simulink model "SolarMicroinverterModelAnalogControl_230V"  (Simulink 8.4)
settings: Solver=ode5  StartTime=0.0  StopTime=0.042  FixedStep=1e-7  RelTol=1e-3
libraries: simulink x2
settings Model: Creator=I14724  LastModifiedBy=ilyas  ParamWorkspaceSource=ReferencedWorkspace  TunableVars=Ts  TunableVarsStorageClass=Auto
settings OptimizationCC: InitFltsAndDblsToZero=on

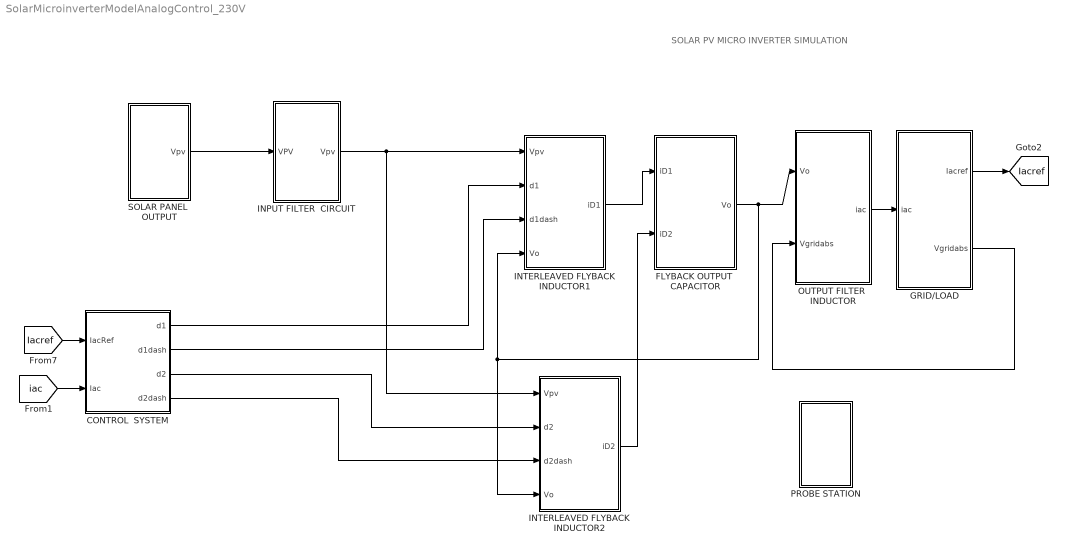
== system SolarMicroinverterModelAnalogControl_230V ==
  note: SOLAR PV MICRO INVERTER SIMULATION
  " CONTROL  SYSTEM" : Subsystem
  FLYBACK OUTPUT  CAPACITOR : Subsystem
  GRID/LOAD : Subsystem
  INPUT FILTER  CIRCUIT : Subsystem
  INTERLEAVED FLYBACK INDUCTOR1 : Subsystem
  INTERLEAVED FLYBACK INDUCTOR2 : Subsystem
  OUTPUT FILTER  INDUCTOR : Subsystem
  PROBE STATION : Subsystem
  SOLAR PANEL  OUTPUT : Subsystem
  tag scope: Iacref=global
  wires:
  INTERLEAVED FLYBACK INDUCTOR1/1(iD1) -> FLYBACK OUTPUT  CAPACITOR/1(iD1)
  FLYBACK OUTPUT  CAPACITOR/1(Vo) -> OUTPUT FILTER  INDUCTOR/1(Vo), INTERLEAVED FLYBACK INDUCTOR2/4(Vo), INTERLEAVED FLYBACK INDUCTOR1/4(Vo)
  OUTPUT FILTER  INDUCTOR/1(iac) -> GRID/LOAD/1(iac)
  GRID/LOAD/2(Vgridabs) -> OUTPUT FILTER  INDUCTOR/2(Vgridabs)
  GRID/LOAD/1(Iacref) -> [Iacref]
  SOLAR PANEL  OUTPUT/1(Vpv) -> INPUT FILTER  CIRCUIT/1(VPV)
  [Iacref] -> " CONTROL  SYSTEM"/1(IacRef)
  [iac] -> " CONTROL  SYSTEM"/2(Iac)
  " CONTROL  SYSTEM"/1(d1) -> INTERLEAVED FLYBACK INDUCTOR1/2(d1)
  " CONTROL  SYSTEM"/2(d1dash) -> INTERLEAVED FLYBACK INDUCTOR1/3(d1dash)
  INPUT FILTER  CIRCUIT/1(Vpv) -> INTERLEAVED FLYBACK INDUCTOR2/1(Vpv), INTERLEAVED FLYBACK INDUCTOR1/1(Vpv)
  " CONTROL  SYSTEM"/3(d2) -> INTERLEAVED FLYBACK INDUCTOR2/2(d2)
  " CONTROL  SYSTEM"/4(d2dash) -> INTERLEAVED FLYBACK INDUCTOR2/3(d2dash)
  INTERLEAVED FLYBACK INDUCTOR2/1(iD2) -> FLYBACK OUTPUT  CAPACITOR/2(iD2)

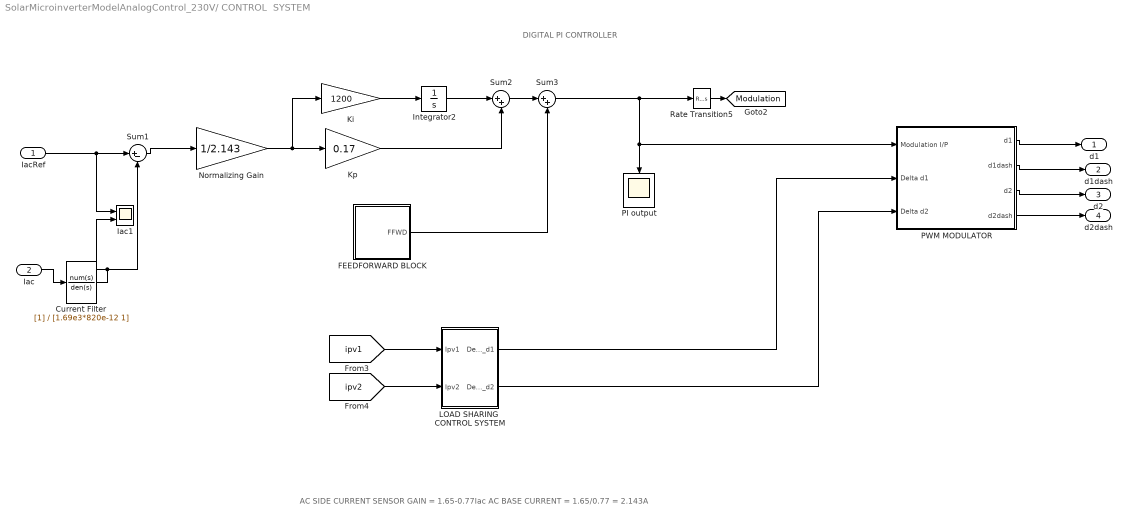
== system SolarMicroinverterModelAnalogControl_230V/ CONTROL  SYSTEM ==
  note: DIGITAL PI CONTROLLER
  note: AC SIDE CURRENT SENSOR GAIN = 1.65-0.77Iac
      | AC BASE CURRENT = 1.65/0.77 = 2.143A
  IacRef : Inport
  Iac : Inport  Port=2
  Current Filter : TransferFcn  Denominator=[1.69e3*820e-12 1]
  FEEDFORWARD BLOCK : Subsystem
  Iac1 : Scope  NumInputPorts=2
      settings: YMin=-5.5~-5.5  YMax=5.5~5.5  SaveName=ScopeData24
  Integrator2 : Integrator
  Ki : Gain  Gain=1200
  Kp : Gain  Gain=0.17
  LOAD SHARING  CONTROL SYSTEM : Subsystem
  Normalizing Gain : Gain  Gain=1/2.143
  PI output : Scope
      settings: TimeRange=0.01  YMin=0.15  YMax=0.5  SaveName=ScopeData15
  PWM MODULATOR : Subsystem
  Rate Transition5 : RateTransition  OutPortSampleTimeOpt=Inherit
  Sum1 : Sum  Inputs=|+-
  Sum2 : Sum  Inputs=|++
  Sum3 : Sum  Inputs=|++
  d1 : Outport
  d1dash : Outport  Port=2
  d2 : Outport  Port=3
  d2dash : Outport  Port=4
  tag scope: Modulation=global
  wires:
  IacRef/1 -> Sum1/1, Iac1/1
  PWM MODULATOR/1(d1) -> d1/1
  PWM MODULATOR/2(d1dash) -> d1dash/1
  Iac/1 -> Current Filter/1
  PWM MODULATOR/3(d2) -> d2/1
  PWM MODULATOR/4(d2dash) -> d2dash/1
  [ipv1] -> LOAD SHARING  CONTROL SYSTEM/1(Ipv1)
  [ipv2] -> LOAD SHARING  CONTROL SYSTEM/2(Ipv2)
  LOAD SHARING  CONTROL SYSTEM/1(Delta_d1) -> PWM MODULATOR/2(Delta d1)
  Rate Transition5/1 -> [Modulation]
  Sum1/1 -> Normalizing Gain/1
  Ki/1 -> Integrator2/1
  Normalizing Gain/1 -> Kp/1, Ki/1
  Sum2/1 -> Sum3/1
  Sum3/1 -> PI output/1, PWM MODULATOR/1(Modulation I/P), Rate Transition5/1
  Integrator2/1 -> Sum2/1
  Kp/1 -> Sum2/2
  FEEDFORWARD BLOCK/1(FFWD) -> Sum3/2
  LOAD SHARING  CONTROL SYSTEM/2(Delta_d2) -> PWM MODULATOR/3(Delta d2)
  Current Filter/1 -> Iac1/2, Sum1/2

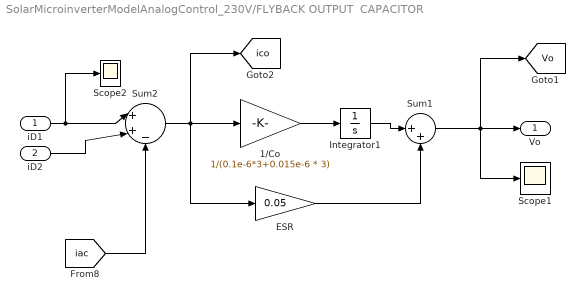
== system SolarMicroinverterModelAnalogControl_230V/FLYBACK OUTPUT  CAPACITOR ==
  iD1 : Inport
  iD2 : Inport  Port=2
  1/Co : Gain  Gain=1/(0.1e-6*3+0.015e-6 * 3)
  ESR : Gain  Gain=0.05
  Integrator1 : Integrator
  Scope1 : Scope
      settings: YMin=-25  YMax=350
  Scope2 : Scope
      settings: YMin=0  YMax=8  SaveName=ScopeData2
  Sum1 : Sum  Inputs=|++
  Sum2 : Sum  Inputs=|++-
  Vo : Outport
  tag scope: Vo=global, ico=global
  wires:
  1/Co/1 -> Integrator1/1
  Sum2/1 -> [ico], 1/Co/1, ESR/1
  Integrator1/1 -> Sum1/1
  Sum1/1 -> Vo/1, [Vo], Scope1/1
  ESR/1 -> Sum1/2
  iD1/1 -> Sum2/1, Scope2/1
  iD2/1 -> Sum2/2
  [iac] -> Sum2/3

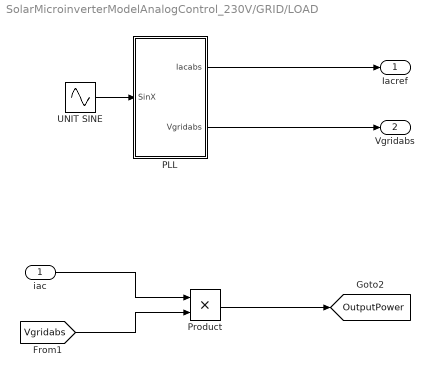
== system SolarMicroinverterModelAnalogControl_230V/GRID/LOAD ==
  iac : Inport
  PLL : Subsystem
  Product : Product  RndMeth=Zero
  UNIT SINE : Sin  Frequency=2*pi*60  SampleTime=0
  Iacref : Outport
  Vgridabs : Outport  Port=2
  tag scope: OutputPower=global
  wires:
  UNIT SINE/1 -> PLL/1(SinX)
  iac/1 -> Product/1
  Product/1 -> [OutputPower]
  [Vgridabs] -> Product/2
  PLL/1(Iacabs) -> Iacref/1
  PLL/2(Vgridabs) -> Vgridabs/1

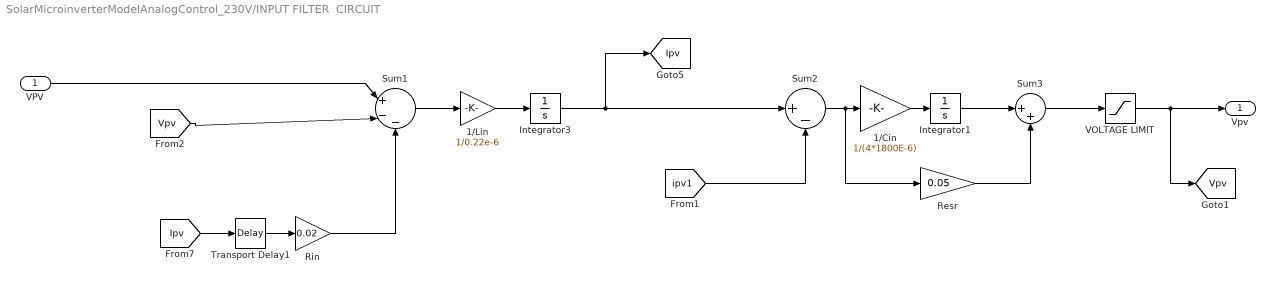
== system SolarMicroinverterModelAnalogControl_230V/INPUT FILTER  CIRCUIT ==
  VPV : Inport
  1/Cin : Gain  Gain=1/(4*1800E-6)
  1/Lin : Gain  Gain=1/0.22e-6
  Integrator1 : Integrator
  Integrator3 : Integrator
  Resr : Gain  Gain=0.05
  Rin : Gain  Gain=0.02
  Sum1 : Sum  Inputs=|+--
  Sum2 : Sum  Inputs=|+-
  Sum3 : Sum  Inputs=|++
  Transport Delay1 : TransportDelay  DelayTime=1e-7
  VOLTAGE LIMIT : Saturate  UpperLimit=100  LowerLimit=0
  Vpv : Outport
  tag scope: Ipv=global, Vpv=global
  wires:
  [ipv1] -> Sum2/2
  Integrator3/1 -> [Ipv], Sum2/1
  [Vpv] -> Sum1/2
  VPV/1 -> Sum1/1
  Rin/1 -> Sum1/3
  Transport Delay1/1 -> Rin/1
  [Ipv] -> Transport Delay1/1
  1/Lin/1 -> Integrator3/1
  Sum1/1 -> 1/Lin/1
  Sum2/1 -> 1/Cin/1, Resr/1
  1/Cin/1 -> Integrator1/1
  VOLTAGE LIMIT/1 -> Vpv/1, [Vpv]
  Integrator1/1 -> Sum3/1
  Sum3/1 -> VOLTAGE LIMIT/1
  Resr/1 -> Sum3/2

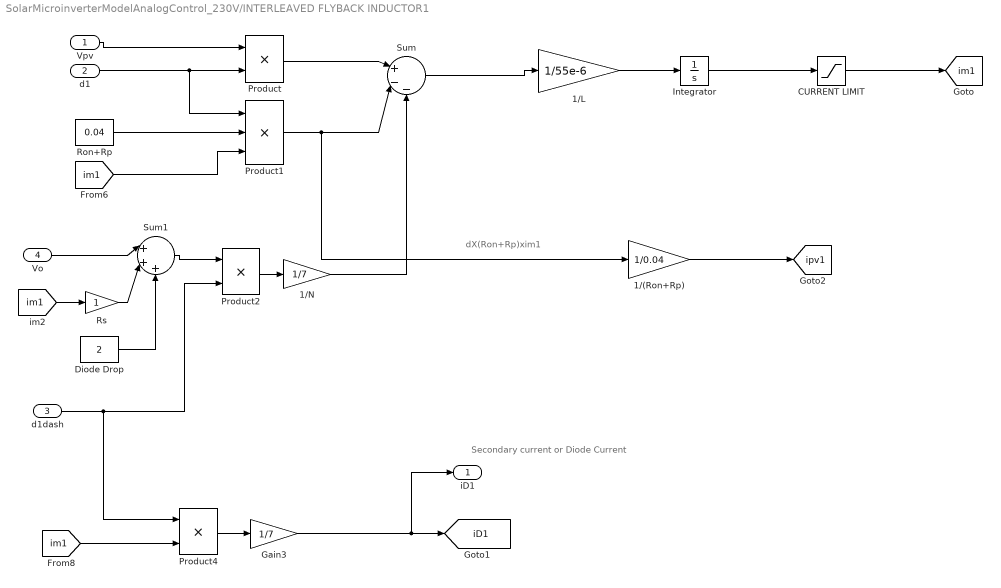
== system SolarMicroinverterModelAnalogControl_230V/INTERLEAVED FLYBACK INDUCTOR1 ==
  note: Secondary current or Diode Current
  note: dX(Ron+Rp)xim1
  Vpv : Inport
  d1 : Inport  Port=2
  d1dash : Inport  Port=3
  Vo : Inport  Port=4
  1/(Ron+Rp) : Gain  Gain=1/0.04
  1/L : Gain  Gain=1/55e-6
  1/N : Gain  Gain=1/7
  CURRENT LIMIT : Saturate  UpperLimit=200  LowerLimit=-1
  Diode Drop : Constant  Value=2
  Gain3 : Gain  Gain=1/7
  Integrator : Integrator
  Product : Product  RndMeth=Zero
  Product1 : Product  Inputs=3  RndMeth=Zero
  Product2 : Product  RndMeth=Zero
  Product4 : Product  RndMeth=Zero
  Ron+Rp : Constant  Value=0.04
  Rs : Gain
  Sum : Sum  Inputs=|+--
  Sum1 : Sum  Inputs=|+++
  iD1 : Outport
  tag scope: iD1=global, im1=global, ipv1=global
  wires:
  Integrator/1 -> CURRENT LIMIT/1
  1/N/1 -> Sum/3
  Product2/1 -> 1/N/1
  Sum1/1 -> Product2/1
  Product1/1 -> Sum/2, 1/(Ron+Rp)/1
  Product/1 -> Sum/1
  d1/1 -> Product/2, Product1/1
  Vpv/1 -> Product/1
  1/L/1 -> Integrator/1
  Sum/1 -> 1/L/1
  CURRENT LIMIT/1 -> [im1]
  [im1] -> Product4/2
  Gain3/1 -> [iD1], iD1/1
  Ron+Rp/1 -> Product1/2
  [im1] -> Product1/3
  Product4/1 -> Gain3/1
  Vo/1 -> Sum1/1
  d1dash/1 -> Product2/2, Product4/1
  1/(Ron+Rp)/1 -> [ipv1]
  [im1] -> Rs/1
  Diode Drop/1 -> Sum1/3
  Rs/1 -> Sum1/2

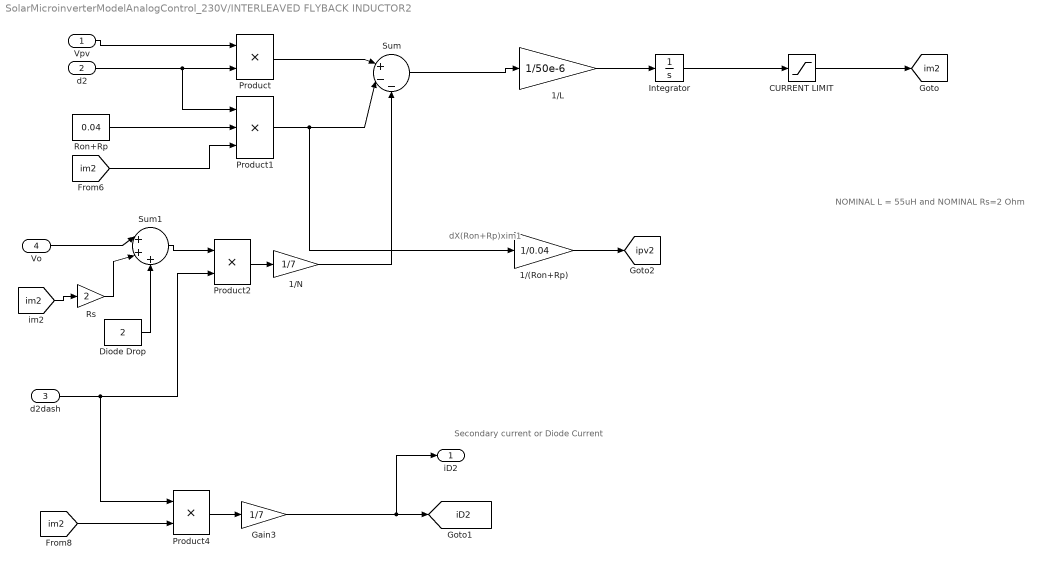
== system SolarMicroinverterModelAnalogControl_230V/INTERLEAVED FLYBACK INDUCTOR2 ==
  note: dX(Ron+Rp)xim1
  note: Secondary current or Diode Current
  note: NOMINAL L = 55uH and NOMINAL Rs=2 Ohm
  Vpv : Inport
  d2 : Inport  Port=2
  d2dash : Inport  Port=3
  Vo : Inport  Port=4
  1/(Ron+Rp) : Gain  Gain=1/0.04
  1/L : Gain  Gain=1/50e-6
  1/N : Gain  Gain=1/7
  CURRENT LIMIT : Saturate  UpperLimit=200  LowerLimit=-1
  Diode Drop : Constant  Value=2
  Gain3 : Gain  Gain=1/7
  Integrator : Integrator
  Product : Product  RndMeth=Zero
  Product1 : Product  Inputs=3  RndMeth=Zero
  Product2 : Product  RndMeth=Zero
  Product4 : Product  RndMeth=Zero
  Ron+Rp : Constant  Value=0.04
  Rs : Gain  Gain=2
  Sum : Sum  Inputs=|+--
  Sum1 : Sum  Inputs=|+++
  iD2 : Outport
  tag scope: iD2=global, im2=global, ipv2=global
  wires:
  1/(Ron+Rp)/1 -> [ipv2]
  d2dash/1 -> Product4/1, Product2/2
  Vo/1 -> Sum1/1
  Product4/1 -> Gain3/1
  [im2] -> Product1/3
  Ron+Rp/1 -> Product1/2
  Gain3/1 -> iD2/1, [iD2]
  [im2] -> Product4/2
  CURRENT LIMIT/1 -> [im2]
  Sum/1 -> 1/L/1
  1/L/1 -> Integrator/1
  Vpv/1 -> Product/1
  d2/1 -> Product1/1, Product/2
  Product/1 -> Sum/1
  Product1/1 -> 1/(Ron+Rp)/1, Sum/2
  [im2] -> Rs/1
  Sum1/1 -> Product2/1
  Product2/1 -> 1/N/1
  1/N/1 -> Sum/3
  Integrator/1 -> CURRENT LIMIT/1
  Rs/1 -> Sum1/2
  Diode Drop/1 -> Sum1/3

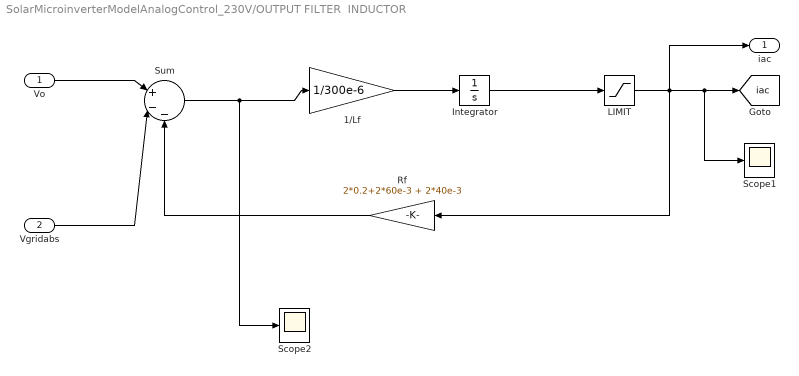
== system SolarMicroinverterModelAnalogControl_230V/OUTPUT FILTER  INDUCTOR ==
  Vo : Inport
  Vgridabs : Inport  Port=2
  " LIMIT" : Saturate  UpperLimit=10  LowerLimit=-0.4
  1/Lf : Gain  Gain=1/300e-6
  Integrator : Integrator
  Rf : Gain  Gain=2*0.2+2*60e-3 + 2*40e-3
  Scope1 : Scope
      settings: YMin=-0.2  YMax=1.2  SaveName=ScopeData8
  Scope2 : Scope
      settings: YMin=-3  YMax=3  SaveName=ScopeData13
  Sum : Sum  Inputs=|+--
  iac : Outport
  tag scope: iac=global
  wires:
  Vgridabs/1 -> Sum/2
  Integrator/1 -> " LIMIT"/1
  Vo/1 -> Sum/1
  1/Lf/1 -> Integrator/1
  Sum/1 -> 1/Lf/1, Scope2/1
  " LIMIT"/1 -> iac/1, Rf/1, [iac], Scope1/1
  Rf/1 -> Sum/3

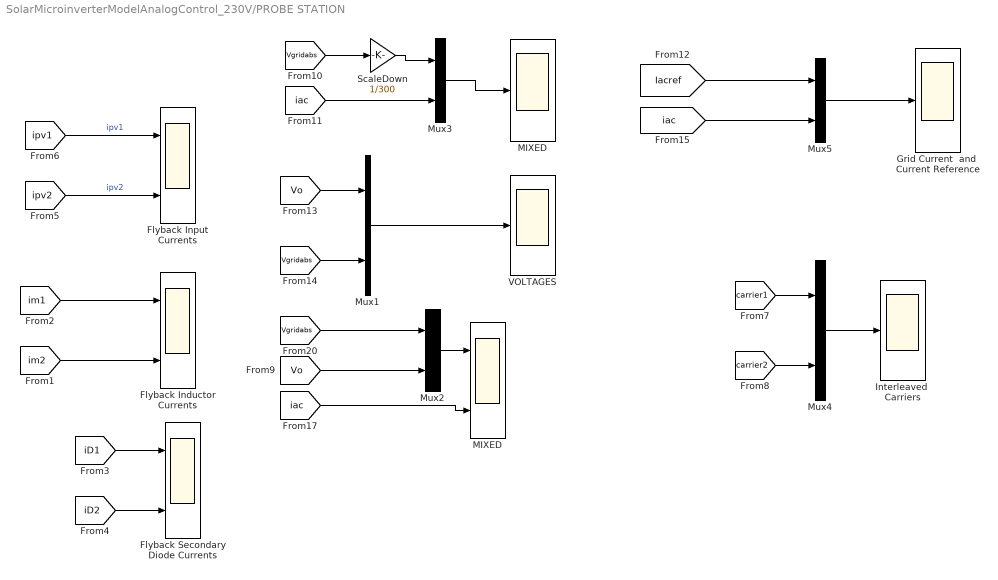
== system SolarMicroinverterModelAnalogControl_230V/PROBE STATION ==
  Flyback Inductor Currents : Scope  NumInputPorts=2
      settings: YMin=280~1.025  YMax=345~1.325
  Flyback Input Currents : Scope  NumInputPorts=2
      settings: YMin=280~1.025  YMax=345~1.325
  Flyback Secondary Diode Currents : Scope  NumInputPorts=2
      settings: YMin=280~1.025  YMax=345~1.325  SaveName=ScopeData2
  Grid Current  and  Current Reference : Scope
      settings: TimeRange=0.03  YMin=0.9  YMax=1.275  SaveName=ScopeData30
  Interleaved  Carriers : Scope
      settings: YMin=0  YMax=1  SaveName=ScopeData6
  MIXED : Scope
      settings: YMin=0.675  YMax=1.2  SaveName=ScopeData27
  "MIXED " : Scope  NumInputPorts=2
      settings: YMin=280~1.025  YMax=345~1.325  SaveName=ScopeData10
  Mux{1..5} (5 alike) : Mux  Inputs=2
  ScaleDown : Gain  Gain=1/300
  "VOLTAGES " : Scope
      settings: YMin=-1000  YMax=1500  SaveName=ScopeData9
  wires:
  [Vo] -> Mux1/1
  [Vgridabs] -> Mux1/2
  Mux1/1 -> "VOLTAGES "/1
  Mux2/1 -> "MIXED "/1
  [Vgridabs] -> Mux2/1
  [Vo] -> Mux2/2
  [iac] -> "MIXED "/2
  [carrier1] -> Mux4/1
  Mux4/1 -> Interleaved  Carriers/1
  [carrier2] -> Mux4/2
  Mux5/1 -> Grid Current  and  Current Reference/1
  [Iacref] -> Mux5/1
  [iac] -> Mux5/2
  [ipv1] -> Flyback Input Currents/1  "ipv1"
  [ipv2] -> Flyback Input Currents/2  "ipv2"
  [im1] -> Flyback Inductor Currents/1
  [im2] -> Flyback Inductor Currents/2
  [iD1] -> Flyback Secondary Diode Currents/1
  [iD2] -> Flyback Secondary Diode Currents/2
  Mux3/1 -> MIXED/1
  [Vgridabs] -> ScaleDown/1
  [iac] -> Mux3/2
  ScaleDown/1 -> Mux3/1

== system SolarMicroinverterModelAnalogControl_230V/SOLAR PANEL  OUTPUT ==
  Vmpp : Constant  Value=36
  Vpv : Outport
  tag scope: VPV=global
  wires:
  Vmpp/1 -> [VPV], Vpv/1

== system SolarMicroinverterModelAnalogControl_230V/ CONTROL  SYSTEM/FEEDFORWARD BLOCK ==
  Divide : Product  Inputs=*/
  Sum4 : Sum  Inputs=|++
  TURNS1 : Gain  Gain=7
  FFWD : Outport
  wires:
  [Vo] -> Sum4/1
  [Vpv] -> TURNS1/1
  [Vo] -> Divide/1
  Sum4/1 -> Divide/2
  TURNS1/1 -> Sum4/2
  Divide/1 -> FFWD/1

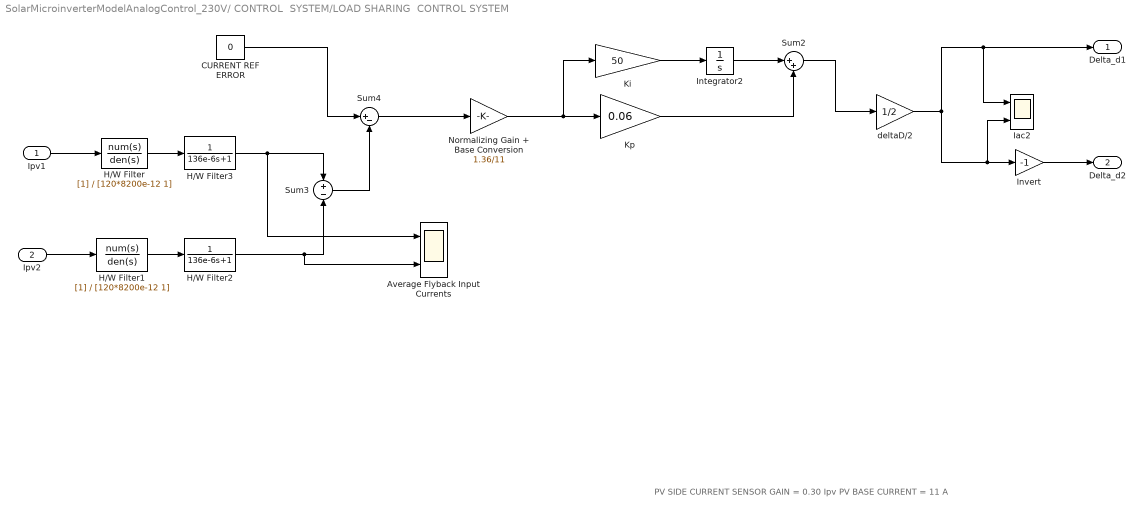
== system SolarMicroinverterModelAnalogControl_230V/ CONTROL  SYSTEM/LOAD SHARING  CONTROL SYSTEM ==
  note: PV SIDE CURRENT SENSOR GAIN = 0.30 Ipv
      | PV BASE CURRENT =  11 A
  Ipv1 : Inport
  Ipv2 : Inport  Port=2
  Average Flyback Input Currents : Scope  NumInputPorts=2
      settings: TimeRange=0.03  YMin=2.8~2.7  YMax=4.9~5  SaveName=ScopeData3
  CURRENT REF ERROR : Constant  Value=0
  H/W Filter : TransferFcn  Denominator=[120*8200e-12 1]
  H/W Filter1 : TransferFcn  Denominator=[120*8200e-12 1]
  H/W Filter2 : TransferFcn  Denominator=[136e-6 1]
  H/W Filter3 : TransferFcn  Denominator=[136e-6 1]
  Iac2 : Scope  NumInputPorts=2
      settings: YMin=0.0015~0.0015  YMax=0.0085~0.0085  SaveName=ScopeData32
  Integrator2 : Integrator  InitialCondition=0.01
  Invert : Gain  Gain=-1
  Ki : Gain  Gain=50
  Kp : Gain  Gain=0.06
  Normalizing Gain + Base Conversion : Gain  Gain=1.36/11
  Sum2 : Sum  Inputs=|++
  Sum3 : Sum  Inputs=+-
  Sum4 : Sum  Inputs=|+-
  deltaD/2 : Gain  Gain=1/2
  Delta_d1 : Outport
  Delta_d2 : Outport  Port=2
  wires:
  Ipv1/1 -> H/W Filter/1
  Ipv2/1 -> H/W Filter1/1
  H/W Filter/1 -> H/W Filter3/1
  H/W Filter1/1 -> H/W Filter2/1
  Sum3/1 -> Sum4/2
  Sum4/1 -> Normalizing Gain + Base Conversion/1
  CURRENT REF ERROR/1 -> Sum4/1
  H/W Filter3/1 -> Sum3/1, Average Flyback Input Currents/1
  H/W Filter2/1 -> Sum3/2, Average Flyback Input Currents/2
  deltaD/2/1 -> Invert/1, Iac2/2, Iac2/1, Delta_d1/1
  Ki/1 -> Integrator2/1
  Normalizing Gain + Base Conversion/1 -> Kp/1, Ki/1
  Integrator2/1 -> Sum2/1
  Kp/1 -> Sum2/2
  Sum2/1 -> deltaD/2/1
  Invert/1 -> Delta_d2/1

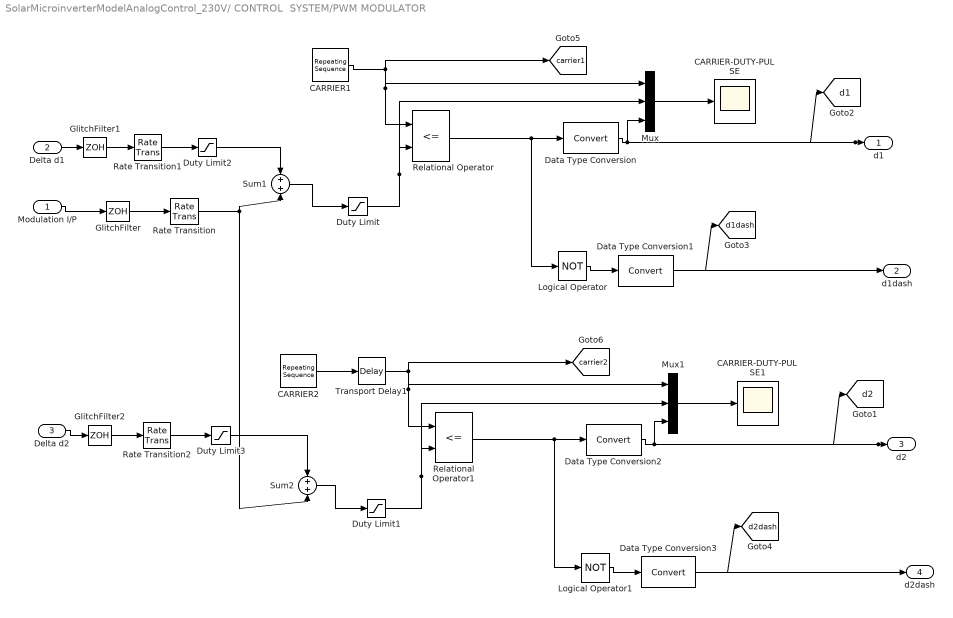
== system SolarMicroinverterModelAnalogControl_230V/ CONTROL  SYSTEM/PWM MODULATOR ==
  Modulation I/P : Inport
  Delta d1 : Inport  Port=2
  Delta d2 : Inport  Port=3
  CARRIER-DUTY-PULSE : Scope
      settings: YMin=0  YMax=1  SaveName=ScopeData28
  CARRIER-DUTY-PULSE1 : Scope
      settings: YMin=0.12  YMax=0.31  SaveName=ScopeData19
  CARRIER1 : simulink/Sources/Repeating Sequence  rep_seq_t=[0 17e-6]  rep_seq_y=[0 1]
  CARRIER2 : simulink/Sources/Repeating Sequence  rep_seq_t=[0 17e-6]  rep_seq_y=[0 1]
  Data Type Conversion{,1..3} (4 alike) : DataTypeConversion
  Duty Limit : Saturate  UpperLimit=0.75  LowerLimit=0
  Duty Limit1 : Saturate  UpperLimit=0.75  LowerLimit=0
  Duty Limit2 : Saturate  UpperLimit=0.02  LowerLimit=0
  Duty Limit3 : Saturate  UpperLimit=0.02  LowerLimit=0
  GlitchFilter : ZeroOrderHold  SampleTime=17e-6
  GlitchFilter1 : ZeroOrderHold  SampleTime=200e-6
  GlitchFilter2 : ZeroOrderHold  SampleTime=200e-6
  Logical Operator : Logic  Operator=NOT  AllPortsSameDT=off  OutDataTypeStr=boolean
  Logical Operator1 : Logic  Operator=NOT  AllPortsSameDT=off  OutDataTypeStr=boolean
  Mux : Mux  Inputs=3
  Mux1 : Mux  Inputs=3
  Rate Transition : RateTransition
  Rate Transition1 : RateTransition
  Rate Transition2 : RateTransition
  Relational Operator : RelationalOperator  Operator=<=  OutDataTypeStr=boolean
  Relational Operator1 : RelationalOperator  Operator=<=  OutDataTypeStr=boolean
  Sum1 : Sum
  Sum2 : Sum
  Transport Delay1 : TransportDelay  DelayTime=8.5e-6
  d1 : Outport
  d1dash : Outport  Port=2
  d2 : Outport  Port=3
  d2dash : Outport  Port=4
  tag scope: carrier1=global, carrier2=global, d1=global, d1dash=global, d2=global, d2dash=global
  wires:
  CARRIER1/1 -> [carrier1], Relational Operator/1, Mux/1
  Relational Operator/1 -> Logical Operator/1, Data Type Conversion/1
  Logical Operator/1 -> Data Type Conversion1/1
  Data Type Conversion/1 -> d1/1, [d1], Mux/3
  Data Type Conversion1/1 -> d1dash/1, [d1dash]
  Modulation I/P/1 -> GlitchFilter/1
  Duty Limit/1 -> Relational Operator/2, Mux/2
  Mux/1 -> CARRIER-DUTY-PULSE/1
  CARRIER2/1 -> Transport Delay1/1
  Relational Operator1/1 -> Data Type Conversion2/1, Logical Operator1/1
  Logical Operator1/1 -> Data Type Conversion3/1
  Data Type Conversion2/1 -> [d2], d2/1, Mux1/3
  Data Type Conversion3/1 -> [d2dash], d2dash/1
  Duty Limit1/1 -> Mux1/2, Relational Operator1/2
  Mux1/1 -> CARRIER-DUTY-PULSE1/1
  Sum1/1 -> Duty Limit/1
  Sum2/1 -> Duty Limit1/1
  Transport Delay1/1 -> Mux1/1, Relational Operator1/1, [carrier2]
  Delta d1/1 -> GlitchFilter1/1
  Delta d2/1 -> GlitchFilter2/1
  Duty Limit2/1 -> Sum1/1
  Duty Limit3/1 -> Sum2/1
  GlitchFilter/1 -> Rate Transition/1
  Rate Transition/1 -> Sum1/2, Sum2/2
  GlitchFilter1/1 -> Rate Transition1/1
  Rate Transition1/1 -> Duty Limit2/1
  GlitchFilter2/1 -> Rate Transition2/1
  Rate Transition2/1 -> Duty Limit3/1

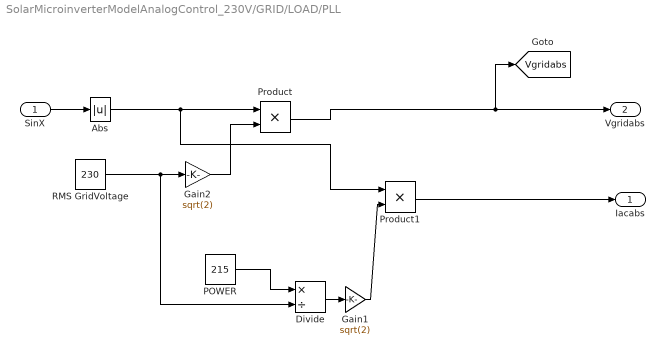
== system SolarMicroinverterModelAnalogControl_230V/GRID/LOAD/PLL ==
  SinX : Inport
  Abs : Abs
  Divide : Product  Inputs=*/
  Gain1 : Gain  Gain=sqrt(2)
  Gain2 : Gain  Gain=sqrt(2)
  POWER : Constant  Value=215
  Product : Product  RndMeth=Zero
  Product1 : Product  RndMeth=Zero
  RMS GridVoltage : Constant  Value=230
  Iacabs : Outport
  Vgridabs : Outport  Port=2
  tag scope: Vgridabs=global
  wires:
  Abs/1 -> Product/1, Product1/1
  SinX/1 -> Abs/1
  Product/1 -> Vgridabs/1, [Vgridabs]
  RMS GridVoltage/1 -> Gain2/1, Divide/2
  Gain2/1 -> Product/2
  POWER/1 -> Divide/1
  Divide/1 -> Gain1/1
  Product1/1 -> Iacabs/1
  Gain1/1 -> Product1/2
